simulink model "FuSimp01"  (Simulink 5.0)
settings: Solver=ode23tb  StartTime=0.0  StopTime=inf  MaxStep=1/90000  MinStep=1/100000000  RelTol=1e-6
undefined symbols (not defined in the file or in its folder): get
libraries: simulink x3, commcontsrc2 x2, dspsnks4 x1
settings Model: LastModifiedBy=efst

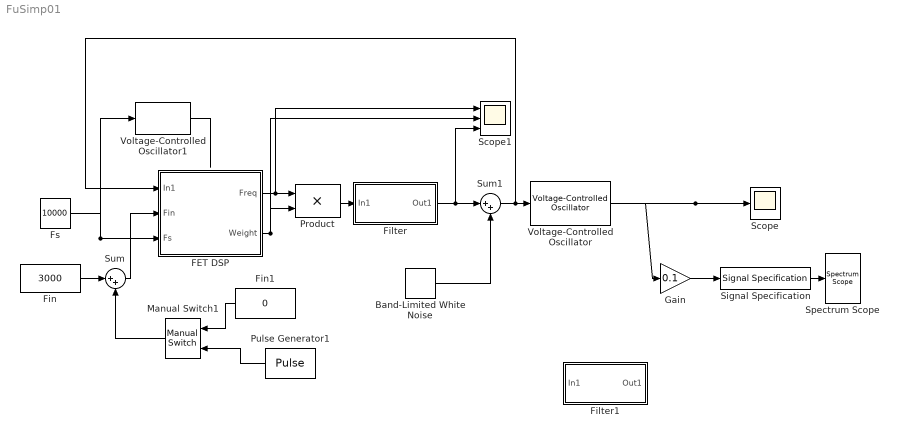
== system FuSimp01 ==
  Band-Limited White Noise : simulink/Sources/Band-Limited White Noise  Cov=[0.001]  Ts=1/10000  seed=[23341]
  FET DSP : Subsystem  TreatAsAtomicUnit=on
  Filter : Subsystem  TreatAsAtomicUnit=on
  Filter1 : Subsystem  TreatAsAtomicUnit=on
  Fin : Constant  Value=3000
  Fin1 : Constant  Orientation=left  Value=0
  Fs : Constant  Value=10000
  Gain : Gain  Gain=0.1  SaturateOnIntegerOverflow=on
  Manual Switch1 : simulink/Signal Routing/Manual Switch  Orientation=left  sw=0  action=0
  Product : Product  SaturateOnIntegerOverflow=on
  Pulse Generator1 : DiscretePulseGenerator  Orientation=left  PulseType=Time based  Amplitude=1000  Period=1/100  PulseWidth=50
  Scope : Scope
      settings: TimeRange=0.0009417969485778867  YMin=-1  YMax=1
  Scope1 : Scope  NumInputPorts=3
      settings: TimeRange=0.02  YMin=-1500~0.95~2500  YMax=1500~1.05~4500
  Signal Specification : simulink/Signal Attributes/Signal Specification  D=1  Ts=1/10000  DataType=auto  OutDataType=sfix(16)  OutScaling=2^0
      settings: SignalType=auto  SamplingMode=sample-based
  Spectrum Scope : dspsnks4/Spectrum Scope  ScopeProperties=on  Domain=Frequency  HorizSpan=1  UseBuffer=on  BufferSize=1024  Overlap=64  inpFftLenInherit=on  FFTlength=1024  numAvg=12  DisplayProperties=off  AxisGrid=on  Memory=off  FrameNumber=on  AxisLegend=off  AxisZoom=off  OpenScopeAtSimStart=on  OpenScopeImmediately=off  FigPos=get(0,'defaultfigureposition')  AxisProperties=off  XUnits=Hertz  XRange=[0...Fs/2]  InheritXIncr=on  XIncr=1.0  XLabel=Samples  YUnits=dB  YLabel=Magnitude, dB  LineProperties=off
      settings: YMin=-96.9843310890135  YMax=7.04988374964699
  Sum : Sum  Inputs=|++  SaturateOnIntegerOverflow=on
  Sum1 : Sum  Inputs=|++  SaturateOnIntegerOverflow=on
  Voltage-Controlled Oscillator : commcontsrc2/Voltage-Controlled Oscillator  Ac=1  Fc=0  Kc=1  Ph=0
  Voltage-Controlled Oscillator1 : commcontsrc2/Voltage-Controlled Oscillator  Ac=1  Fc=0  Kc=1  Ph=0
  wires:
  Fs/1 -> FET DSP/3(Fs), Voltage-Controlled Oscillator1/1
  Voltage-Controlled Oscillator1/1 -> ?
  Signal Specification/1 -> Spectrum Scope/1
  FET DSP/1(Freq) -> Product/1, Scope1/1
  FET DSP/2(Weight) -> Product/2, Scope1/2
  Voltage-Controlled Oscillator/1 -> Scope/1, Gain/1
  Fin/1 -> Sum/1
  Manual Switch1/1 -> Sum/2
  Sum/1 -> FET DSP/2(Fin)
  Pulse Generator1/1 -> Manual Switch1/2
  Fin1/1 -> Manual Switch1/1
  Sum1/1 -> Voltage-Controlled Oscillator/1, FET DSP/1(In1)
  Band-Limited White Noise/1 -> Sum1/2
  Gain/1 -> Signal Specification/1
  Product/1 -> Filter/1(In1)
  Filter/1(Out1) -> Sum1/1, Scope1/3

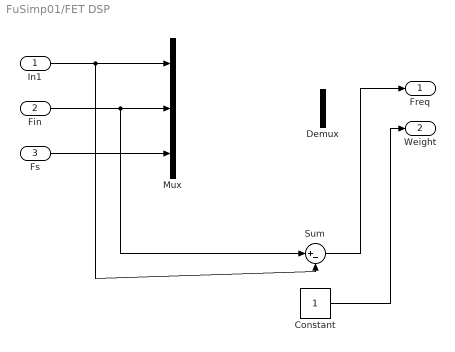
== system FuSimp01/FET DSP ==
  In1 : Inport
  Fin : Inport  Port=2
  Fs : Inport  Port=3
  Constant : Constant
  Demux : Demux  Outputs=2
  Mux : Mux  Inputs=3
  Sum : Sum  Inputs=|+-  SaturateOnIntegerOverflow=on
  Freq : Outport
  Weight : Outport  Port=2
  wires:
  Fin/1 -> Mux/2, Sum/1
  In1/1 -> Mux/1, Sum/2
  Fs/1 -> Mux/3
  ? -> Demux/1
  Sum/1 -> Freq/1
  Constant/1 -> Weight/1

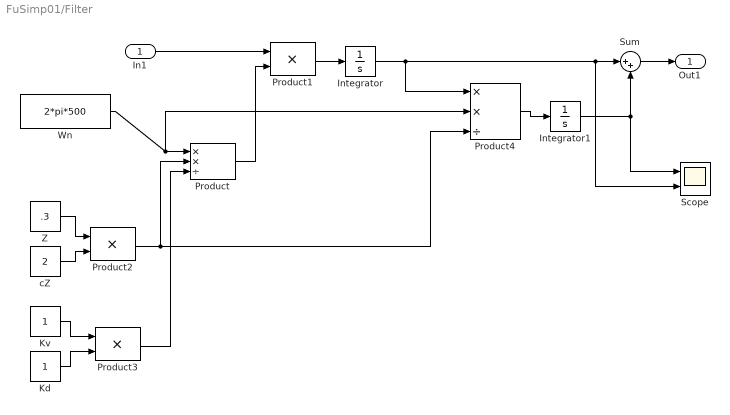
== system FuSimp01/Filter ==
  In1 : Inport
  Integrator : Integrator  UpperSaturationLimit=10  LowerSaturationLimit=-10
  Integrator1 : Integrator  InitialCondition=100  LimitOutput=on  UpperSaturationLimit=5000  LowerSaturationLimit=100
  Kd : Constant
  Kv : Constant
  Product : Product  Inputs=**/  ShowAdditionalParam=on  RndMeth=Nearest  SaturateOnIntegerOverflow=on
  Product1 : Product  SaturateOnIntegerOverflow=on
  Product2 : Product  SaturateOnIntegerOverflow=on
  Product3 : Product  SaturateOnIntegerOverflow=on
  Product4 : Product  Inputs=**/  SaturateOnIntegerOverflow=on
  Scope : Scope  NumInputPorts=2
      settings: TimeRange=0.01  YMin=2000~-1000  YMax=3000~1000  SaveName=ScopeData2
  Sum : Sum  Inputs=|++  SaturateOnIntegerOverflow=on
  Wn : Constant  Value=2*pi*500
  Z : Constant  Value=.3
  cZ : Constant  Value=2
  Out1 : Outport
  wires:
  Product/1 -> Product1/2
  Z/1 -> Product2/1
  cZ/1 -> Product2/2
  Product2/1 -> Product/2, Product4/3
  Kv/1 -> Product3/1
  Kd/1 -> Product3/2
  Wn/1 -> Product/1, Product4/2
  Product3/1 -> Product/3
  Product1/1 -> Integrator/1
  Sum/1 -> Out1/1
  Integrator/1 -> Product4/1, Sum/1, Scope/2
  In1/1 -> Product1/1
  Product4/1 -> Integrator1/1
  Integrator1/1 -> Sum/2, Scope/1

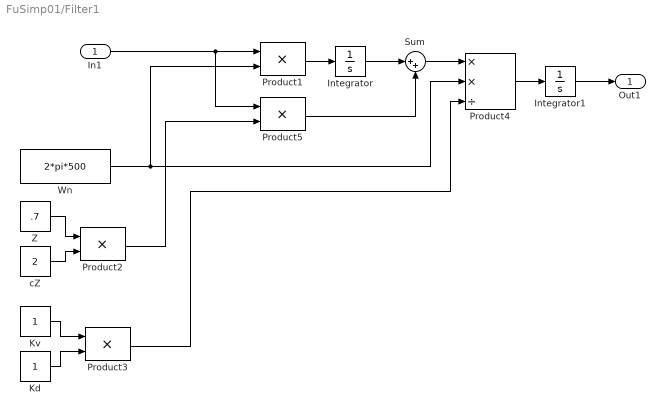
== system FuSimp01/Filter1 ==
  In1 : Inport
  Integrator : Integrator  UpperSaturationLimit=10  LowerSaturationLimit=-10  ZeroCross=off
  Integrator1 : Integrator  InitialCondition=1000  LimitOutput=on  UpperSaturationLimit=5000  LowerSaturationLimit=100
  Kd : Constant
  Kv : Constant
  Product{1..3,5} (4 alike) : Product  SaturateOnIntegerOverflow=on
  Product4 : Product  Inputs=**/  SaturateOnIntegerOverflow=on
  Sum : Sum  Inputs=|++  SaturateOnIntegerOverflow=on
  Wn : Constant  Value=2*pi*500
  Z : Constant  Value=.7
  cZ : Constant  Value=2
  Out1 : Outport
  wires:
  Z/1 -> Product2/1
  cZ/1 -> Product2/2
  Kv/1 -> Product3/1
  Kd/1 -> Product3/2
  Wn/1 -> Product1/2, Product4/2
  Product1/1 -> Integrator/1
  In1/1 -> Product1/1, Product5/1
  Integrator/1 -> Sum/1
  Product2/1 -> Product5/2
  Product5/1 -> Sum/2
  Sum/1 -> Product4/1
  Product3/1 -> Product4/3
  Product4/1 -> Integrator1/1
  Integrator1/1 -> Out1/1
